simulink model "verify_Velocity_mdl"  (R2013b)
settings: Solver=VariableStepDiscrete  StartTime=0.0  StopTime=10.0  MaxStep=0.1  RelTol=1e-3
libraries: carnot x2
settings Model: Creator=drhf  LastModifiedBy=drhf
settings OptimizationCC: ExpressionDepthLimit=2147483647
settings DebuggingCC: StateNameClashWarn=warning
settings GRTTargetCC: CombineOutputUpdateFcns=off  GRTInterface=on

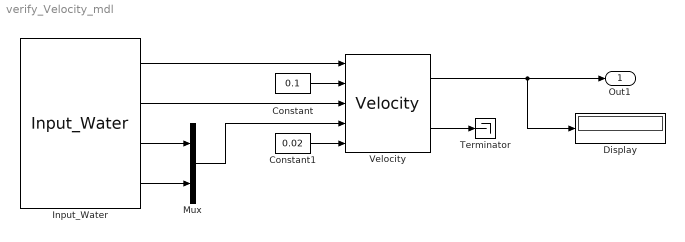
== system verify_Velocity_mdl ==
  Constant : Constant  Value=0.1
  Constant1 : Constant  Value=0.02
  Display : Display
  Input_Water : carnot/Basic/Material_Properties/Input_Water  T=20  p=2e6  xd=0
  Mux : Mux  Inputs=2
  Terminator : Terminator
  Velocity : carnot/Basic/Hydraulics/Velocity
  Out1 : Outport
  wires:
  Input_Water/2 -> Velocity/3
  Input_Water/1 -> Velocity/1
  Input_Water/4 -> Mux/2
  Input_Water/3 -> Mux/1
  Velocity/1 -> Display/1, Out1/1
  Mux/1 -> Velocity/4
  Constant/1 -> Velocity/2
  Constant1/1 -> Velocity/5
  Velocity/2 -> Terminator/1
